simulink model "AdaptiveControl"  (R2024a)
settings: Solver=ode5  StartTime=0.0  StopTime=10  FixedStep=0.0001  MaxStep=0.01  RelTol=1e-3
InitFcn:
  | params
values from neighbouring files (symbols this model uses):
  am = 1/(Rlnom*C)    (= 53.1914893617)    [params.m]
  bm = 1    [params.m]
  C = 470e-6    (= 0.00047)    [params.m]
  eta_d = 10    [params.m]
  eta_q = 8    [params.m]
  k1 = 5000000    [params.m]
  k2 = 400000    [params.m]
  k3 = 700000    [params.m]
  kappa = 320    [params.m]
  L = 0.5e-3    (= 0.0005)    [params.m]
  lambbda_d = 2900    [params.m]
  lambda_q = 20    [params.m]
  omega = 100*pi    (= 314.159265359)    [params.m]
  Qas = bm    (= 1)    [params.m]
  R = 0.1    [params.m]
  Rlnom = 40    [params.m]
  Thetaas = 0    [params.m]
  vod = 200    [params.m]
undefined symbols (not defined in the file or in its folder): dspblkCoreblockFVToolHelper, gcbh
libraries: simulink x3, slpidlib x1
settings Model: Creator=gerardo.flores  LastModifiedBy=gerardo.flores
settings SolverCC: ZeroCrossControl=EnableAll

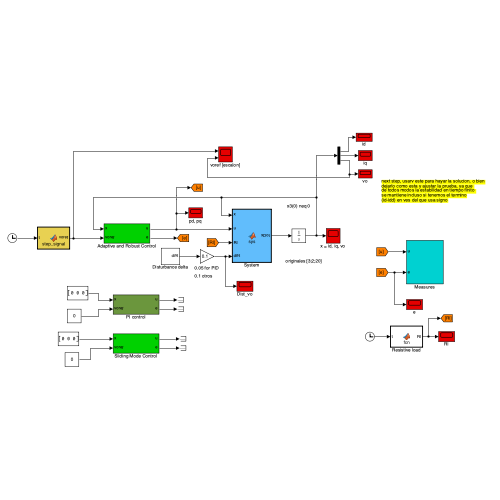
[thumbnail: Simulink's stored preview of the top-level diagram]
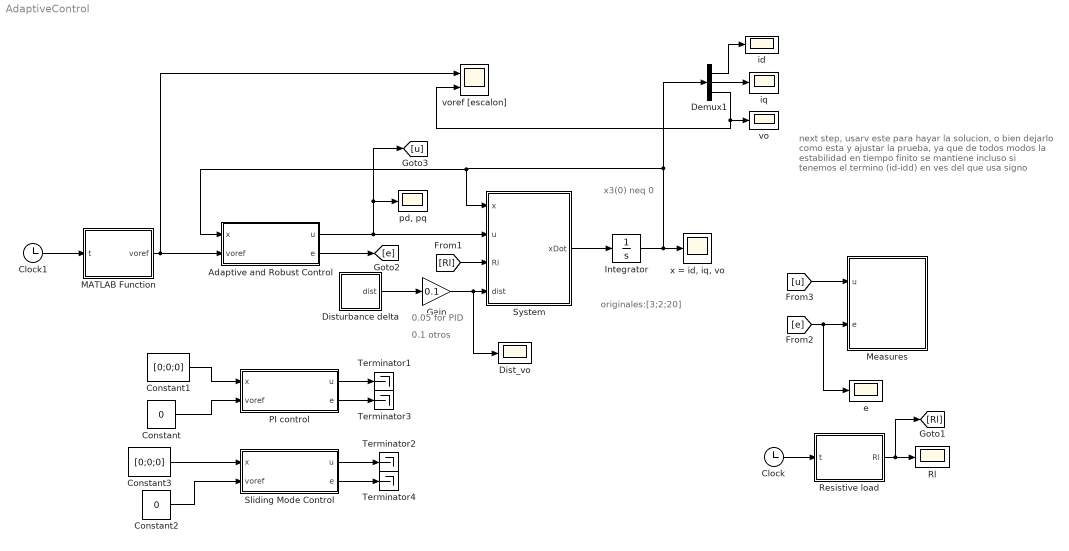
== system AdaptiveControl ==
  note: 0.1 otros
  note: 0.05 for PID
  note: originales:[3;2;20]
  note: next step, usarv este para hayar la solucion, o bien
      | dejarlo como esta y ajustar la prueba, ya que
      | de todos modos la estabilidad en tiempo finito
      | se mantiene incluso si tenemos el termino
      | (id-idd) en ves del que usa signo
  note: x3(0) neq 0
  Adaptive and Robust Control : Subsystem
  Clock : Clock
  Clock1 : Clock
  Constant : Constant  Value=0
  Constant1 : Constant  Value=[0;0;0]
  Constant2 : Constant  Value=0
  Constant3 : Constant  Value=[0;0;0]
  Demux1 : Demux  Outputs=3
  Dist_vo : Scope
  Disturbance delta : Subsystem
  Gain : Gain  Gain=0.1
  Integrator : Integrator  InitialCondition=[30;20;20]
  MATLAB Function : MATLAB Function  TreatAsAtomicUnit=on
  Measures : Subsystem
  PI control : Subsystem
  Resistive load : MATLAB Function  TreatAsAtomicUnit=on
  Rl : Scope
  Sliding Mode Control : Subsystem
  System : MATLAB Function  TreatAsAtomicUnit=on
  Terminator{1..4} (4 alike) : Terminator
  e : Scope
  id : Scope
  iq : Scope
  "pd, pq" : Scope
  vo : Scope
  voref [escalon] : Scope  NumInputPorts=2
  "x = id, iq, vo" : Scope
  wires:
  System/1(xDot) -> Integrator/1
  Integrator/1 -> "x = id, iq, vo"/1, Demux1/1, Adaptive and Robust Control/1(x), System/1(x)
  Demux1/1 -> id/1
  Demux1/2 -> iq/1
  Demux1/3 -> voref [escalon]/2, vo/1
  Adaptive and Robust Control/1(u) -> [u], "pd, pq"/1, System/2(u)
  [Rl] -> System/3(Rl)
  Clock/1 -> Resistive load/1(t)
  Resistive load/1(Rl) -> [Rl], Rl/1
  Disturbance delta/1(dist) -> Gain/1
  MATLAB Function/1(voref) -> Adaptive and Robust Control/2(voref), voref [escalon]/1
  Clock1/1 -> MATLAB Function/1(t)
  PI control/1(u) -> Terminator1/1
  Constant1/1 -> PI control/1(x)
  Constant/1 -> PI control/2(voref)
  Gain/1 -> Dist_vo/1, System/4(dist)
  Sliding Mode Control/1(u) -> Terminator2/1
  Constant3/1 -> Sliding Mode Control/1(x)
  Constant2/1 -> Sliding Mode Control/2(voref)
  Adaptive and Robust Control/2(e) -> [e]
  [u] -> Measures/1(u)
  [e] -> e/1, Measures/2(e)
  PI control/2(e) -> Terminator3/1
  Sliding Mode Control/2(e) -> Terminator4/1

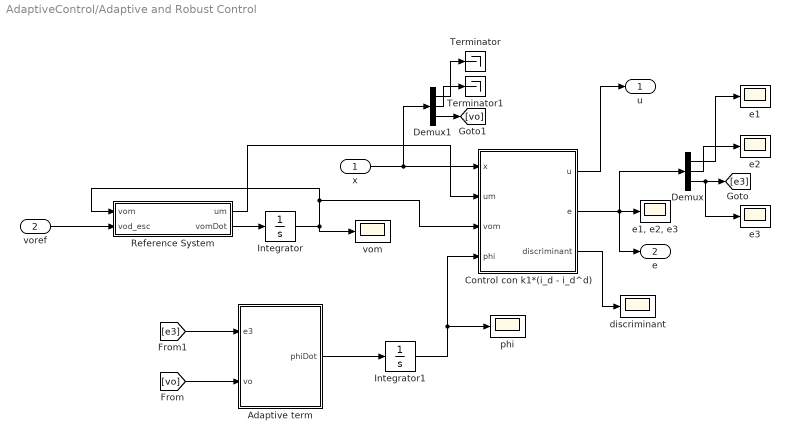
== system AdaptiveControl/Adaptive and Robust Control ==
  x : Inport
  voref : Inport  Port=2
  " e1" : Scope
  " e2" : Scope
  " e3" : Scope
  Adaptive term : MATLAB Function  TreatAsAtomicUnit=on
  Control con k1*(i_d - i_d^d) : MATLAB Function  TreatAsAtomicUnit=on
  Demux : Demux  Outputs=3
  Demux1 : Demux  Outputs=3
  Integrator : Integrator
  Integrator1 : Integrator
  Reference System : MATLAB Function  TreatAsAtomicUnit=on
  Terminator : Terminator
  Terminator1 : Terminator
  discriminant : Scope
  "e1, e2, e3" : Scope
  phi : Scope
  vom : Scope
  u : Outport
  e : Outport  Port=2
  wires:
  x/1 -> Demux1/1, Control con k1*(i_d - i_d^d)/1(x)
  Control con k1*(i_d - i_d^d)/3(discriminant) -> discriminant/1
  Control con k1*(i_d - i_d^d)/2(e) -> e/1, Demux/1, "e1, e2, e3"/1
  Control con k1*(i_d - i_d^d)/1(u) -> u/1
  Reference System/2(vomDot) -> Integrator/1
  Integrator/1 -> vom/1, Reference System/1(vom), Control con k1*(i_d - i_d^d)/3(vom)
  Adaptive term/1(phiDot) -> Integrator1/1
  Reference System/1(um) -> Control con k1*(i_d - i_d^d)/2(um)
  Integrator1/1 -> phi/1, Control con k1*(i_d - i_d^d)/4(phi)
  Demux/3 -> " e3"/1, [e3]
  Demux1/3 -> [vo]
  [e3] -> Adaptive term/1(e3)
  [vo] -> Adaptive term/2(vo)
  Demux1/1 -> Terminator/1
  Demux1/2 -> Terminator1/1
  voref/1 -> Reference System/2(vod_esc)
  Demux/1 -> " e1"/1
  Demux/2 -> " e2"/1

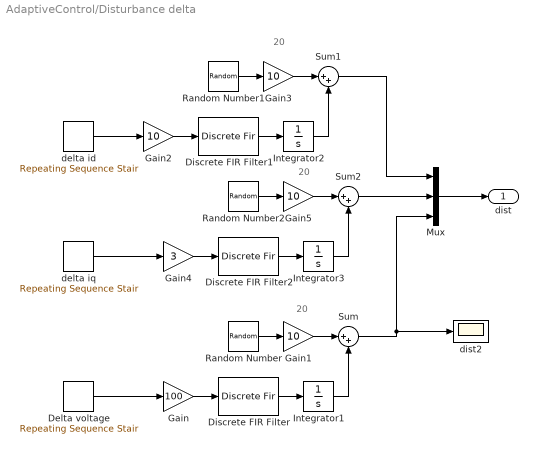
== system AdaptiveControl/Disturbance delta ==
  note: 20
  note: 20
  note: 20
  Delta voltage : simulink/Sources/Repeating Sequence Stair  OutValues=[0 0 1 1 -1 2 -5 -5 -4 1 5 6 7 4].'  tsamp=0.5  OutMin=[]  OutMax=[]  OutDataTypeStr=double  OutputDataTypeScalingMode=double  OutDataType=fixdt(0,8)  ConRadixGroup=Best Precision: Vector-wise  OutScaling=2^-12
  Discrete FIR Filter : DiscreteFir  LoadFcn=dspblkCoreblockFVToolHelper(gcbh,'load');  Coefficients=[1/5 1/5 1/5 1/5 1/5]
      settings: CopyFcn=dspblkCoreblockFVToolHelper(gcbh,'copy');  DeleteFcn=dspblkCoreblockFVToolHelper(gcbh,'close');  ModelCloseFcn=dspblkCoreblockFVToolHelper(gcbh,'close');  PreSaveFcn=dspblkCoreblockFVToolHelper(gcbh,'presave');  PostSaveFcn=dspblkCoreblockFVToolHelper(gcbh,'postsave');  CloseFcn=dspblkCoreblockFVToolHelper(gcbh,'close');
  Discrete FIR Filter1 : DiscreteFir  LoadFcn=dspblkCoreblockFVToolHelper(gcbh,'load');  Coefficients=[1/5 1/5 1/5 1/5 1/5]
      settings: CopyFcn=dspblkCoreblockFVToolHelper(gcbh,'copy');  DeleteFcn=dspblkCoreblockFVToolHelper(gcbh,'close');  ModelCloseFcn=dspblkCoreblockFVToolHelper(gcbh,'close');  PreSaveFcn=dspblkCoreblockFVToolHelper(gcbh,'presave');  PostSaveFcn=dspblkCoreblockFVToolHelper(gcbh,'postsave');  CloseFcn=dspblkCoreblockFVToolHelper(gcbh,'close');
  Discrete FIR Filter2 : DiscreteFir  LoadFcn=dspblkCoreblockFVToolHelper(gcbh,'load');  Coefficients=[1/5 1/5 1/5 1/5 1/5]
      settings: CopyFcn=dspblkCoreblockFVToolHelper(gcbh,'copy');  DeleteFcn=dspblkCoreblockFVToolHelper(gcbh,'close');  ModelCloseFcn=dspblkCoreblockFVToolHelper(gcbh,'close');  PreSaveFcn=dspblkCoreblockFVToolHelper(gcbh,'presave');  PostSaveFcn=dspblkCoreblockFVToolHelper(gcbh,'postsave');  CloseFcn=dspblkCoreblockFVToolHelper(gcbh,'close');
  Gain : Gain  Gain=100
  Gain{1..3,5} (4 alike) : Gain  Gain=10
  Gain4 : Gain  Gain=3
  Integrator1 : Integrator
  Integrator2 : Integrator
  Integrator3 : Integrator
  Mux : Mux  Inputs=3
  Random Number : RandomNumber  SampleTime=0.01
  Random Number1 : RandomNumber  SampleTime=0.01
  Random Number2 : RandomNumber  SampleTime=0.01
  Sum : Sum  Inputs=|++
  Sum1 : Sum  Inputs=|++
  Sum2 : Sum  Inputs=|++
  delta id : simulink/Sources/Repeating Sequence Stair  OutValues=[-3 -4 -7 -7 -1 2 5 5 4 6 3 2 1 0].'  tsamp=0.5  OutMin=[]  OutMax=[]  OutDataTypeStr=double  OutputDataTypeScalingMode=double  OutDataType=fixdt(0,8)  ConRadixGroup=Best Precision: Vector-wise  OutScaling=2^-12
  delta iq : simulink/Sources/Repeating Sequence Stair  OutValues=[1 2 3 4 4 4 5 5 4 4 3 3 3 3].'  tsamp=0.5  OutMin=[]  OutMax=[]  OutDataTypeStr=double  OutputDataTypeScalingMode=double  OutDataType=fixdt(0,8)  ConRadixGroup=Best Precision: Vector-wise  OutScaling=2^-12
  dist2 : Scope
  dist : Outport
  wires:
  Random Number/1 -> Gain1/1
  Delta voltage/1 -> Gain/1
  Gain/1 -> Discrete FIR Filter/1
  Gain1/1 -> Sum/1
  Integrator1/1 -> Sum/2
  Discrete FIR Filter/1 -> Integrator1/1
  Integrator2/1 -> Sum1/2
  Random Number1/1 -> Gain3/1
  delta id/1 -> Gain2/1
  Gain2/1 -> Discrete FIR Filter1/1
  Discrete FIR Filter1/1 -> Integrator2/1
  Gain3/1 -> Sum1/1
  Integrator3/1 -> Sum2/2
  Random Number2/1 -> Gain5/1
  delta iq/1 -> Gain4/1
  Gain4/1 -> Discrete FIR Filter2/1
  Discrete FIR Filter2/1 -> Integrator3/1
  Gain5/1 -> Sum2/1
  Sum2/1 -> Mux/2
  Sum1/1 -> Mux/1
  Sum/1 -> dist2/1, Mux/3
  Mux/1 -> dist/1

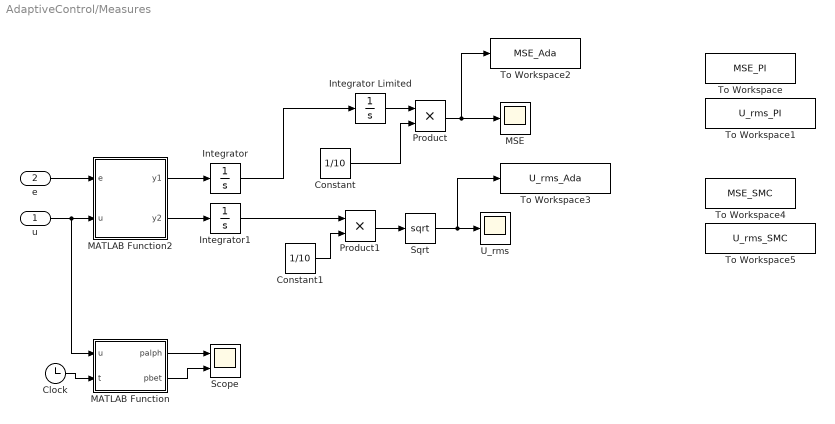
== system AdaptiveControl/Measures ==
  u : Inport
  e : Inport  Port=2
  Clock : Clock
  Constant : Constant  Value=1/10
  Constant1 : Constant  Value=1/10
  Integrator : Integrator
  Integrator Limited : Integrator  UpperSaturationLimit=1  LowerSaturationLimit=0
  Integrator1 : Integrator
  MATLAB Function : MATLAB Function  TreatAsAtomicUnit=on
  MATLAB Function2 : MATLAB Function  TreatAsAtomicUnit=on
  MSE : Scope
  Product : Product
  Product1 : Product
  Scope : Scope  NumInputPorts=2
  Sqrt : Sqrt
  To Workspace : ToWorkspace  VariableName=MSE_PI  SaveFormat=Timeseries  SampleTime=-1
  To Workspace1 : ToWorkspace  VariableName=U_rms_PI  SaveFormat=Timeseries  SampleTime=-1
  To Workspace2 : ToWorkspace  VariableName=MSE_Ada  SaveFormat=Timeseries  SampleTime=-1
  To Workspace3 : ToWorkspace  VariableName=U_rms_Ada  SaveFormat=Timeseries  SampleTime=-1
  To Workspace4 : ToWorkspace  VariableName=MSE_SMC  SaveFormat=Timeseries  SampleTime=-1
  To Workspace5 : ToWorkspace  VariableName=U_rms_SMC  SaveFormat=Timeseries  SampleTime=-1
  U_rms : Scope
  wires:
  Integrator Limited/1 -> Product/1
  Constant/1 -> Product/2
  Product/1 -> To Workspace2/1, MSE/1
  Sqrt/1 -> To Workspace3/1, U_rms/1
  MATLAB Function2/2(y2) -> Integrator1/1
  Constant1/1 -> Product1/2
  Product1/1 -> Sqrt/1
  u/1 -> MATLAB Function/1(u), MATLAB Function2/2(u)
  e/1 -> MATLAB Function2/1(e)
  MATLAB Function2/1(y1) -> Integrator/1
  Integrator/1 -> Integrator Limited/1
  Integrator1/1 -> Product1/1
  Clock/1 -> MATLAB Function/2(t)
  MATLAB Function/1(palph) -> Scope/1
  MATLAB Function/2(pbet) -> Scope/2

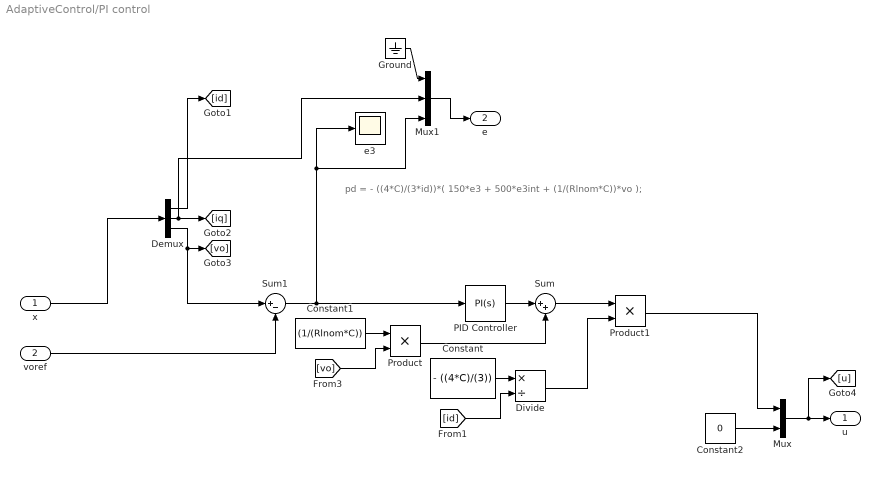
== system AdaptiveControl/PI control ==
  note: pd = - ((4*C)/(3*id))*( 150*e3 + 500*e3int + (1/(Rlnom*C))*vo );
  x : Inport
  voref : Inport  Port=2
  Constant : Constant  Value=- ((4*C)/(3))
  Constant1 : Constant  Value=(1/(Rlnom*C))
  Constant2 : Constant  Value=0
  Demux : Demux  Outputs=3
  Divide : Product  Inputs=*/
  Ground : Ground
  Mux : Mux  Inputs=2
  Mux1 : Mux  Inputs=3
  PID Controller : slpidlib/PID Controller  Controller=PI  Form=Parallel  TimeDomain=Continuous-time  UseExternalTs=off  SampleTime=-1  IntegratorMethod=Forward Euler  FilterMethod=Forward Euler  ControllerParametersSource=internal  P=575.870686369171  I=145933.586108114  UseKiTs=off  D=10  UseExternalDerivativeSource=off  N=100  UseFilter=on  TunerSelectOption=Transfer Function Based (PID Tuner App)  InitialConditionSource=internal  InitialConditionForIntegrator=0  InitialConditionForFilter=0  DifferentiatorICPrevScaledInput=0  ExternalReset=none  TrackingMode=off  Kt=1  LimitOutput=off  SatLimitsSource=internal  UpperSaturationLimit=inf  LowerSaturationLimit=-inf  LinearizeAsGain=on  AntiWindupMode=none  Kb=1  LimitIntegrator=off  UpperIntegratorSaturationLimit=inf  LowerIntegratorSaturationLimit=-inf  POutMin=[]  POutMax=[]  IOutMin=[]  IOutMax=[]  DOutMin=[]  DOutMax=[]  NOutMin=[]  NOutMax=[]  SumOutMin=[]  SumOutMax=[]  SaturationOutMin=[]  SaturationOutMax=[]  PParamMin=[]  PParamMax=[]  IParamMin=[]  IParamMax=[]  DParamMin=[]  DParamMax=[]  NParamMin=[]  NParamMax=[]  KbParamMin=[]  KbParamMax=[]  KtParamMin=[]  KtParamMax=[]  KbOutMin=[]  KbOutMax=[]  KtOutMin=[]  KtOutMax=[]  IntegratorOutMin=[]  IntegratorOutMax=[]  FilterOutMin=[]  FilterOutMax=[]  SumI1OutMin=[]  SumI1OutMax=[]  SumI2OutMin=[]  SumI2OutMax=[]  SumI3OutMin=[]  SumI3OutMax=[]  SumI4OutMin=[]  SumI4OutMax=[]  SumDOutMin=[]  SumDOutMax=[]  DifferentiatorOutMin=[]  DifferentiatorOutMax=[]  FilterDiffOutCoefMin=[]  FilterDiffOutCoefMax=[]  ReciprocalOutMin=[]  ReciprocalOutMax=[]  SumDenOutMin=[]  SumDenOutMax=[]  SumNumOutMin=[]  SumNumOutMax=[]  DivideOutMin=[]  DivideOutMax=[]  UdiffTsProdOutMin=[]  UdiffTsProdOutMax=[]  NTsProdOutMin=[]  NTsProdOutMax=[]  UintegralTsProdOutMin=[]  UintegralTsProdOutMax=[]  UngainTsProdOutMin=[]  UngainTsProdOutMax=[]  ClampingZeroOutDataTypeStr=Inherit: Inherit via back propagation  ClampingZeroOutMin=[]  ClampingZeroOutMax=[]  FilterDenConstantOutDataTypeStr=Inherit: Inherit via back propagation  FilterDenConstantOutMin=[]  FilterDenConstantOutMax=[]  PCopyOutDataTypeStr=Inherit: Inherit via back propagation  PCopyOutMin=[]  PCopyOutMax=[]  NCopyOutDataTypeStr=Inherit: Inherit via back propagation  NCopyOutMin=[]  NCopyOutMax=[]  IntegratorContinuousStateAttributes=''  IntegratorStateMustResolveToSignalObject=off  IntegratorRTWStateStorageClass=Auto  FilterContinuousStateAttributes=''  FilterStateMustResolveToSignalObject=off  FilterRTWStateStorageClass=Auto  ParallelPVariant=InternalParameters  IdealPVariant=Disabled  IVariant=InternalParameters  DVariant=Disabled  IntegratorVariant=Continuous  SatVariant=Disabled  AWVariant=Passthrough  PCopyVariant=Disabled  TRVariant=Disabled  FdbkBlocksVariant=Forward  IdealPFdbkVariant=Disabled  SatFdbkVariant=Disabled  DerivativeFilterVariant=Disabled  NVariant=Disabled  NCopyVariant=Disabled_SignalSpec  FilterICVariant=Disabled  IntegratorICVariant=InternalICs  ExternalResetVariant=Disabled  TRSumVariant=Passthrough  SumFdbkVariant=Disabled  SumVariant=Sum_PI  TsampFilterVariant=InternalTs  TsampNgainVariant=Passthrough  TsampIntegralVariant=Disabled_SignalSpec  ExternalSaturationOutDataTypeStr=Inherit: Same as second input  DerivativeSourceVariant=Disabled
  Product : Product
  Product1 : Product
  Sum : Sum  Inputs=|++
  Sum1 : Sum  Inputs=|+-
  e3 : Scope
  u : Outport
  e : Outport  Port=2
  wires:
  x/1 -> Demux/1
  Mux/1 -> [u], u/1
  Constant/1 -> Divide/1
  Demux/1 -> [id]
  Constant1/1 -> Product/1
  Product/1 -> Sum/2
  Sum/1 -> Product1/1
  Divide/1 -> Product1/2
  Product1/1 -> Mux/1
  [id] -> Divide/2
  Demux/3 -> Sum1/1, [vo]
  [vo] -> Product/2
  Demux/2 -> Mux1/2, [iq]
  Constant2/1 -> Mux/2
  voref/1 -> Sum1/2
  Mux1/1 -> e/1
  Ground/1 -> Mux1/1
  PID Controller/1 -> Sum/1
  Sum1/1 -> Mux1/3, e3/1, PID Controller/1

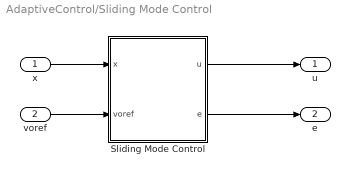
== system AdaptiveControl/Sliding Mode Control ==
  x : Inport
  voref : Inport  Port=2
  Sliding Mode Control : MATLAB Function  TreatAsAtomicUnit=on
  u : Outport
  e : Outport  Port=2
  wires:
  x/1 -> Sliding Mode Control/1(x)
  voref/1 -> Sliding Mode Control/2(voref)
  Sliding Mode Control/1(u) -> u/1
  Sliding Mode Control/2(e) -> e/1

== matlab function AdaptiveControl/Sliding Mode Control/Sliding Mode Control ==
  data: x input; u output; R parameter; L parameter; C parameter; Rlnom parameter; omega parameter; E parameter; voref input; e output; lambbda_d parameter; eta_d parameter; lambda_q parameter; eta_q parameter
function [u, e] = ctrl(x, R, L, C, Rlnom, omega, E, voref, lambbda_d, eta_d, lambda_q, eta_q)

id = x(1,1);
iq = x(2,1); 
vo = x(3,1);

% Errors
e2 = iq;        e3 = vo - voref;

% Controls
%pq = - ( (2*L)/vo )*( (R/L)*iq + omega*id + 2000*e2 + k2smc*sign(e2) )   ;
%pd = (4*C)/(3*id) * (  - pq*iq + (1/(Rlnom*C))*vo - k3smc*sign(e3)  ) ;
pq =  ( (2*L)/vo )*( - (R/L)*iq - omega*id + lambda_q*e2 + eta_q*sign(e2) ) ;
pd = (4*C)/(3*id) * ( (1/(Rlnom*C))*vo - lambbda_d*(e3) - eta_d*sign(e3)  ) ;


% Salidas
u = [pd;
     pq];

e = [ 0;
     e2;
     e3];

== matlab function AdaptiveControl/Measures/MATLAB Function ==
  data: u input; palph output; t input; pbet output; omega parameter
function [palph, pbet] = fcn(u, t, omega)

pd = u(1,1);
pq = u(2,1);

theta = omega*t;

A = [ cos(theta), sin(theta);
     -sin(theta), cos(theta)];


a = A*[pd;pq];

palph = a(1,1);
pbet = a(2,1);

== matlab function AdaptiveControl/Measures/MATLAB Function2 ==
  data: e input; y1 output; u input; y2 output
function [y1, y2] = fcn(e, u)

e1 = e(1,1);
e2 = e(2,1);
e3 = e(3,1);

pd = u(1,1);
pq = u(2,1);

y1 = e2^2 + e3^2;
y2 = pd^2 + pq^2;

== matlab function AdaptiveControl/Adaptive and Robust Control/Reference System ==
  data: um output; vom input; vomDot output; am parameter; bm parameter; kappa parameter; vod_esc input
function [um, vomDot] = ref(vom, am, bm, kappa, vod_esc)

% Control
um = (1/bm)*( am*vom - kappa*(vom - vod_esc) );

% System
vomDot = - am*vom + bm*um ;

== matlab function AdaptiveControl/System ==
  data: x input; u input; Rl input; dist input; R parameter; xDot output; L parameter; C parameter; omega parameter; E parameter
function xDot = sys(x, u, Rl, dist, R, L, C, omega, E)

pd = u(1,1);
pq = u(2,1);

id = x(1,1);
iq = x(2,1); 
vo = x(3,1);

delta_id = dist(1,1);
delta_iq = dist(2,1);
delta_vo = dist(3,1);

% System
idDot = - (R/L)*id - (1/(2*L))*pd*vo + omega*iq + (E/L) + 0*delta_id ;
iqDot = - (R/L)*iq - (1/(2*L))*pq*vo - omega*id + 0*delta_iq ;
voDot = (3/(4*C))*(pd*id + pq*iq) - (1/(Rl*C))*vo + delta_vo/C ;

xDot = [idDot;
        iqDot;
        voDot];

== matlab function AdaptiveControl/Adaptive and Robust Control/Control con k1*(i_d - i_d^d) ==
  data: x input; um input; vom input; phi input; u output; k1 parameter; k2 parameter; k3 parameter; vod parameter; R parameter; L parameter; C parameter; Rlnom parameter; omega parameter; E parameter; e output; discriminant output; Thetaas parameter; Qas parameter
function [u, e, discriminant] = ctrl(x, um, vom, phi, k1, k2, k3, vod, R, L, C, Rlnom, omega, E, Thetaas, Qas)

id = x(1,1);
iq = x(2,1); 
vo = x(3,1);

% Errors e2, e3
e2 = iq;        e3 = vo - vom;
Theta = phi + Thetaas;

% Controls [Adaptive terms]
pq = ( (2*L)/(e3 + vom) )*( - (R/L)*iq - omega*id + k2*e2 ) ; % k2*e2 , k2*sqrt(abs(e2))*sign(e2)
v2 = Theta*vo + Qas*um  - (3/(4*C))*(iq*pq) - k3*e3 ;  % k3*e3 , k3*sqrt(abs(e3))*sign(e3)
%
%pq = ( 2*L/vo )*( - (R/L)*iq - omega*id + k2*sqrt(abs(e2))*sign(e2) ) ; % k2*e2 , k2*sqrt(abs(e2))*sign(e2)
%v2 = - (3/(4*C))*(iq*pq) + (1/(Rl*C))*vo - k3*sqrt(abs(e3))*sign(e3) ;  % k3*e3 , k3*sqrt(abs(e3))*sign(e3)

% Combinando las sigs. eqs (23) [version no adaptiva]
% pd = ((2*L)/(vo)) * ( - (R/L)*id + omega*iq + (E/L) + k1*(id - idd) ) ;
% idd = (4*C*v2)/(3*pd) ; 
% obtenemos:

a = k1;
b = (R/L) * id - omega * iq - (E/L) - k1 * id;
c = (2 * C * v2 * vo) / (3 * L);
discriminant = b^2 - 4 * a * c; %no debe ser cero

idd = ( -b + sqrt(b^2 - 4 * a * c) ) / (2 * a); %id deseada dinamica

pd = (4 * C * v2) / (3 * idd); %sale de (23)------------------> CONTROL REAL

% Error e1
e1 = id - idd;


% Salidas
u = [pd;
     pq];

e = [e1;
     e2;
     e3];

== matlab function AdaptiveControl/Adaptive and Robust Control/Adaptive term ==
  data: e3 input; phiDot output; vo input; lambda parameter
function phiDot = fcn(e3, vo, lambda)


phiDot = - lambda*e3*vo;

== matlab function AdaptiveControl/Resistive load ==
  data: Rl output; Rlnom parameter; t input
function Rl = fcn(Rlnom, t)

Rl = Rlnom + 30*sin(1.5*t);

== matlab function AdaptiveControl/MATLAB Function ==
  data: t input; voref output; vod parameter
function voref = step_signal(t, vod)
% Generates a step signal increasing from 160 to 220 in steps of 20
% over a simulation time of 0 to 10 seconds.

    % Define step times and corresponding values
    %step_times = [0, 3.3, 6.6, 10]; % Change points
    %step_values = [vod-40, vod-20, vod, vod]; % Corresponding values
    step_times = [0, 2, 4, 6, 8]; % Change points
    %step_values = [vod-40, vod-20, vod, vod+20, vod+40]; % Corresponding values
    step_values = [vod, vod+20, vod+40, vod+80, vod+40]; % Corresponding values
    
    % Initialize output
    voref = step_values(1);
    
    % Apply step changes
    for i = 2:length(step_times)
        if t >= step_times(i)
            voref = step_values(i);
        end
    end
end
